simulink model "system_sim"  (R2015a)
settings: Solver=ode45  StartTime=0.0  StopTime=3600 *10  FixedStep=0.2  RelTol=0.001
values from neighbouring files (symbols this model uses):
  area = 1.2    [run_sim_auto.m]    (also in run_sim_test4.m = 2; sim_testing.m; wrkspc_no_1.mat; wrkspc_no_10.mat)
  Cd = 0.6    [run_sim_auto.m]    (also in run_sim_test4.m = 1; sim_testing.m; wrkspc_no_1.mat; wrkspc_no_10.mat)
  Crr = 0.005    [run_sim_test4.m]    (also in wrkspc_no_1.mat; wrkspc_no_10.mat; wrkspc_no_18.mat; wrkspc_no_22.mat)
  eff_vals = eff_data(:,2)    [run_sim_auto.m]    (also in wrkspc_no_1.mat = [5.2 10.3 15.5 20.6 25.8 31 36.1 41.3 46.4 51.6 56.8 61.9 ..; wrkspc_no_10.mat = [5.2 10.3 15.5 20.6 25.8 31 36.1 41.3 46.4 51.6 56.8 61.9 ..; wrkspc_no_18.mat = [5.2 10.3 15.5 20.6 25.8 31 36.1 41.3 46.4 51.6 56.8 61.9 ..; wrkspc_no_22.mat = [5.2 10.3 15.5 20.6 25.8 31 36.1 41.3 46.4 51.6 56.8 61.9 ..)
  end_x = x_in_m(length(x_in_m))    [run_sim_auto.m]    (also in run_sim_v2.m; wrkspc_no_1.mat = 44100; wrkspc_no_10.mat = 48084; wrkspc_no_18.mat = 8912)
  fmax = max_moving_force    [run_sim_auto.m]    (also in run_sim_v2.m; wrkspc_no_1.mat = 666.666666667; wrkspc_no_10.mat = 666.666666667; wrkspc_no_18.mat = 666.666666667)
  g = 9.81    [run_sim.m]    (also in run_sim_auto.m; run_sim_test.m; run_sim_test4.m; run_sim_v2.m)
  input_rpm_vals = eff_data(:,1)    [run_sim_auto.m]    (also in wrkspc_no_1.mat = [10 20 30 40 50 60 70 80 90 100 110 120 ... (35 elements, 35; wrkspc_no_10.mat = [10 20 30 40 50 60 70 80 90 100 110 120 ... (35 elements, 35; wrkspc_no_18.mat = [10 20 30 40 50 60 70 80 90 100 110 120 ... (35 elements, 35; wrkspc_no_22.mat = [10 20 30 40 50 60 70 80 90 100 110 120 ... (35 elements, 35)
  m = 210    [run_sim_auto.m]    (also in run_sim_test4.m = 150; sim_testing.m; wrkspc_no_1.mat; wrkspc_no_10.mat)
  rho_air = 1.225    [run_sim.m]    (also in run_sim_auto.m; run_sim_test.m; run_sim_test4.m; run_sim_v2.m)
  slope = target_speed_m_s/acc_time    [run_sim_auto.m]    (also in run_sim_v2.m; wrkspc_no_1.mat = 0.833333333333; wrkspc_no_10.mat = 0.833333333333; wrkspc_no_18.mat = 0.833333333333)
  target_speed_m_s = 4.16    [run_sim_test4.m]    (also in wrkspc_no_1.mat = 4.16666666667; wrkspc_no_10.mat = 4.16666666667; wrkspc_no_18.mat = 4.16666666667; wrkspc_no_22.mat = 4.16666666667)
  wheel_radius = 0.2538    [wrkspc_no_1.mat]    (also in wrkspc_no_10.mat; wrkspc_no_18.mat; wrkspc_no_22.mat)
libraries: simulink x1
settings Model: Creator=marco  LastModifiedBy=marco

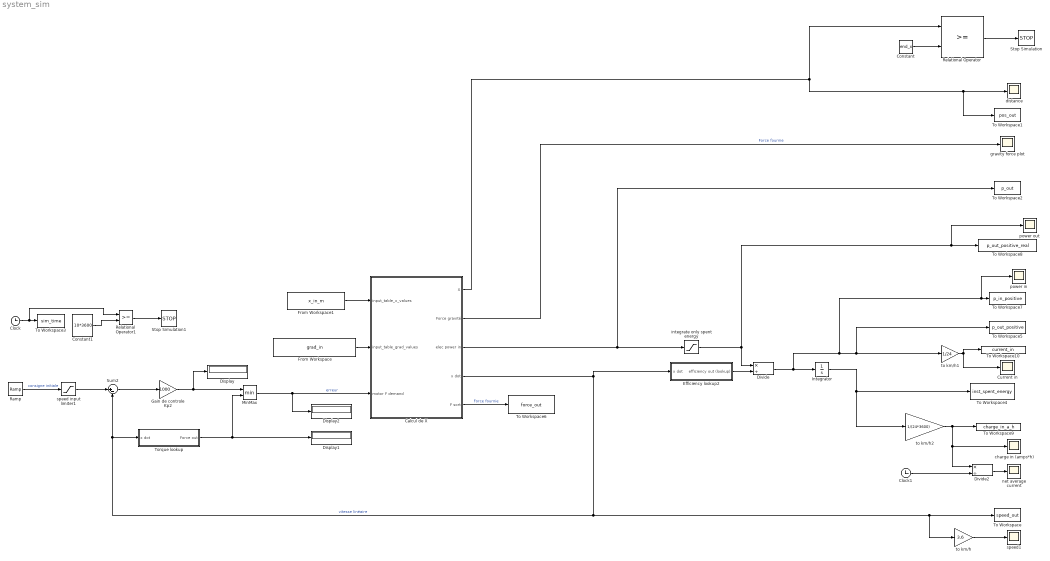
== system system_sim ==
  Calcul de X : Subsystem
  Clock : Clock
  Clock1 : Clock
  Constant : Constant  Value=end_x
  Constant1 : Constant  Value=10*3600
  Current in : Scope
      settings: TimeRange=10000  YMin=0  YMax=40  SaveName=ScopeData5  MaxDataPoints=scope_history*3
  Display : Display
  Display1 : Display
  Display2 : Display
  Divide : Product  Inputs=*/
  Divide2 : Product  Inputs=*/
  Efficiency lookup2 : Subsystem
  From Workspace : FromWorkspace  VariableName=grad_in  SampleTime=0
  From Workspace1 : FromWorkspace  VariableName=x_in_m  SampleTime=0
  Gain de controle Kp2 : Gain  Gain=1000
  Integrator : Integrator
  MinMax : MinMax  Inputs=2
  Ramp : simulink/Sources/Ramp  slope=slope  start=0  X0=0
  Relational Operator : RelationalOperator  OutDataTypeStr=boolean
  Relational Operator1 : RelationalOperator  OutDataTypeStr=boolean
  Stop Simulation : Stop
  Stop Simulation1 : Stop
  Sum2 : Sum  Inputs=|+-
  To Workspace : ToWorkspace  VariableName=speed_out  SampleTime=-1
      settings: Save2DSignal=2-D array (concatenate along first dimension)
  To Workspace1 : ToWorkspace  VariableName=pos_out  SampleTime=-1
      settings: Save2DSignal=2-D array (concatenate along first dimension)
  To Workspace10 : ToWorkspace  VariableName=current_in  SampleTime=-1
      settings: Save2DSignal=2-D array (concatenate along first dimension)
  To Workspace2 : ToWorkspace  VariableName=p_out  SampleTime=-1
      settings: Save2DSignal=2-D array (concatenate along first dimension)
  To Workspace3 : ToWorkspace  VariableName=sim_time  SampleTime=-1
      settings: Save2DSignal=2-D array (concatenate along first dimension)
  To Workspace4 : ToWorkspace  VariableName=inst_spent_energy  SampleTime=-1
      settings: Save2DSignal=2-D array (concatenate along first dimension)
  To Workspace5 : ToWorkspace  VariableName=p_out_positive  SampleTime=-1
      settings: Save2DSignal=2-D array (concatenate along first dimension)
  To Workspace6 : ToWorkspace  VariableName=force_out  SampleTime=-1
      settings: Save2DSignal=2-D array (concatenate along first dimension)
  To Workspace7 : ToWorkspace  VariableName=p_in_positive  SampleTime=-1
      settings: Save2DSignal=2-D array (concatenate along first dimension)
  To Workspace8 : ToWorkspace  VariableName=p_out_positive_real  SampleTime=-1
      settings: Save2DSignal=2-D array (concatenate along first dimension)
  To Workspace9 : ToWorkspace  VariableName=charge_in_a_h  SampleTime=-1
      settings: Save2DSignal=2-D array (concatenate along first dimension)
  Torque lookup : Subsystem
  charge in (amps*h) : Scope
      settings: TimeRange=30000  YMin=160000  YMax=300000  SaveName=ScopeData7  MaxDataPoints=scope_history *3
  distance : Scope
      settings: YMin=25000  YMax=52500  MaxDataPoints=scope_history
  gravity force plot : Scope
      settings: YMin=3.55  YMax=4.45  MaxDataPoints=scope_history
  integrate only spent energy : Saturate  UpperLimit=fmax*target_speed_m_s*8  LowerLimit=0
  net average current : Scope
      settings: TimeRange=10000  YMin=0  YMax=40  SaveName=ScopeData11  MaxDataPoints=scope_history*3
  power in : Scope
      settings: YMin=0  YMax=425  SaveName=powerin_scope  MaxDataPoints=scope_history*3
  power out : Scope
      settings: YMin=0  YMax=525  SaveName=powerin_scope1  MaxDataPoints=scope_history*3
  speed input limiter1 : Saturate  UpperLimit=target_speed_m_s  LowerLimit=0
  speed1 : Scope
      settings: YMin=7  YMax=15.5  SaveName=speed_kmh_scope  MaxDataPoints=scope_history*3
  to km/h : Gain  Gain=3.6
  to km/h1 : Gain  Gain=1/24
  to km/h2 : Gain  Gain=1/(24*3600)
  wires:
  From Workspace1/1 -> Calcul de X/1(input_table_x_values)
  From Workspace/1 -> Calcul de X/2(input_table_grad_values)
  MinMax/1 -> Calcul de X/3(motor F demand), Display2/1  "erreur"
  Calcul de X/1(X) -> To Workspace1/1, distance/1, Relational Operator/1
  Constant/1 -> Relational Operator/2
  Relational Operator/1 -> Stop Simulation/1
  Clock/1 -> Relational Operator1/1, To Workspace3/1
  Integrator/1 -> to km/h2/1, To Workspace4/1
  integrate only spent energy/1 -> Divide/1, power out/1, To Workspace8/1
  Calcul de X/3(elec power in) -> To Workspace2/1, integrate only spent energy/1
  Constant1/1 -> Relational Operator1/2
  Relational Operator1/1 -> Stop Simulation1/1
  to km/h/1 -> speed1/1
  Calcul de X/5(F sort) -> To Workspace6/1  "Force fournie"
  Ramp/1 -> speed input limiter1/1  "consigne initiale"
  Gain de controle Kp2/1 -> Display/1, MinMax/1
  Sum2/1 -> Gain de controle Kp2/1
  Efficiency lookup2/1(efficiency out (lookup)) -> Divide/2
  Divide/1 -> Integrator/1, power in/1, To Workspace7/1, to km/h1/1, To Workspace5/1
  Calcul de X/4(x dot) -> Sum2/2, Torque lookup/1(x dot), To Workspace/1, to km/h/1, Efficiency lookup2/1(x dot)  "vitesse linéaire"
  speed input limiter1/1 -> Sum2/1
  to km/h1/1 -> Current in/1, To Workspace10/1
  to km/h2/1 -> To Workspace9/1, Divide2/1, charge in (amps*h)/1
  Clock1/1 -> Divide2/2
  Divide2/1 -> net average current/1
  Calcul de X/2(Force gravité) -> gravity force plot/1  "Force fournie"
  Torque lookup/1(Force out) -> MinMax/2, Display1/1

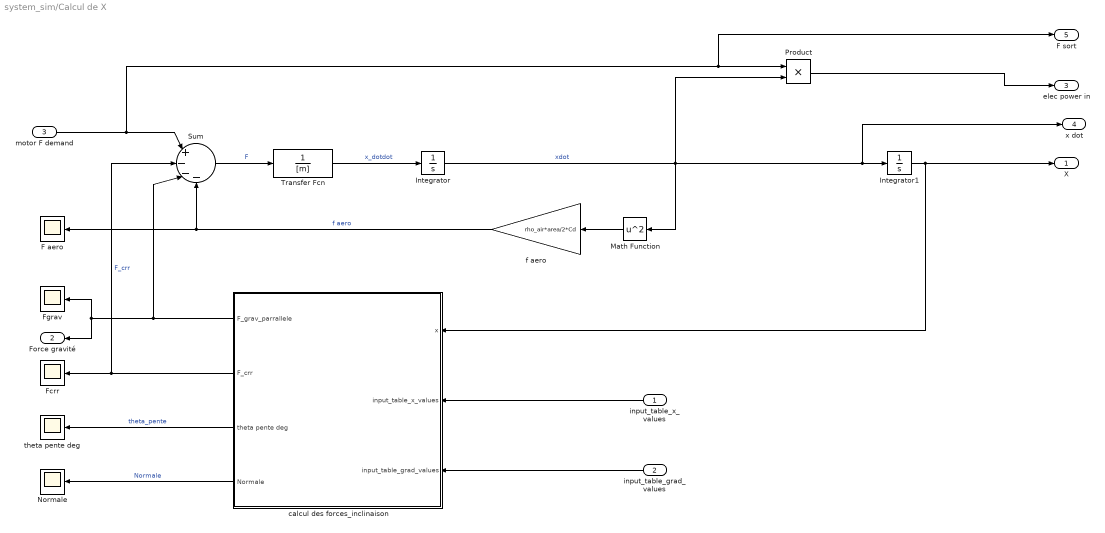
== system system_sim/Calcul de X ==
  input_table_x_values : Inport
  input_table_grad_values : Inport  Port=2
  motor F demand : Inport  Port=3
  F aero : Scope
      settings: SaveName=ScopeData14  MaxDataPoints=scope_history
  Fcrr : Scope
      settings: SaveName=ScopeData10  MaxDataPoints=scope_history
  Fgrav : Scope
      settings: YMin=-70  YMax=70  SaveName=ScopeData9  MaxDataPoints=scope_history*3
  Integrator : Integrator
  Integrator1 : Integrator
  Math Function : Math  Operator=square  SaturateOnIntegerOverflow=on
  Normale : Scope
      settings: SaveName=ScopeData2  MaxDataPoints=scope_history
  Product : Product
  Sum : Sum  Inputs=|+---
  Transfer Fcn : TransferFcn  Denominator=[m]
  calcul des forces_inclinaison : Subsystem
  f aero : Gain  Gain=rho_air*area/2*Cd
  "theta pente deg " : Scope
      settings: YMin=-15  YMax=17.5  SaveName=gradiant  MaxDataPoints=scope_history*3
  X : Outport
  Force gravité : Outport  Port=2
  elec power in : Outport  Port=3
  x dot : Outport  Port=4
  F sort : Outport  Port=5
  wires:
  Sum/1 -> Transfer Fcn/1  "F"
  Transfer Fcn/1 -> Integrator/1  "x_dotdot"
  Integrator/1 -> Math Function/1, Product/2, x dot/1, Integrator1/1  "xdot"
  f aero/1 -> F aero/1, Sum/4  "f aero"
  input_table_x_values/1 -> calcul des forces_inclinaison/2(input_table_x_values)
  input_table_grad_values/1 -> calcul des forces_inclinaison/3(input_table_grad_values)
  Math Function/1 -> f aero/1
  Integrator1/1 -> X/1, calcul des forces_inclinaison/1(x)
  calcul des forces_inclinaison/3(theta pente deg) -> "theta pente deg "/1  "theta_pente"
  calcul des forces_inclinaison/2(F_crr) -> Sum/2, Fcrr/1  "F_crr"
  calcul des forces_inclinaison/1(F_grav_parrallele) -> Sum/3, Force gravité/1, Fgrav/1
  calcul des forces_inclinaison/4(Normale) -> Normale/1  "Normale"
  Product/1 -> elec power in/1
  motor F demand/1 -> Sum/1, F sort/1, Product/1

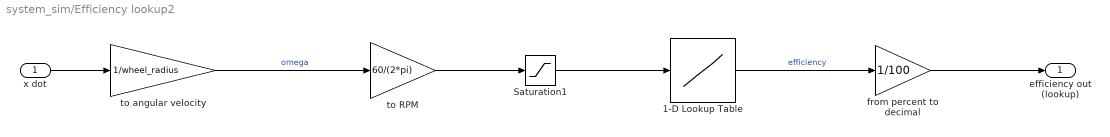
== system system_sim/Efficiency lookup2 ==
  x dot : Inport
  1-D Lookup Table : Lookup_n-D  NumberOfTableDimensions=1  BreakpointsForDimension1=input_rpm_vals  Table=eff_vals  InternalRulePriority=Speed  RndMeth=Simplest  InputSameDT=on
  Saturation1 : Saturate  UpperLimit=177  LowerLimit=10
  from percent to decimal : Gain  Gain=1/100
  to RPM : Gain  Gain=60/(2*pi)
  to angular velocity : Gain  Gain=1/wheel_radius
  efficiency out (lookup) : Outport
  wires:
  x dot/1 -> to angular velocity/1
  to angular velocity/1 -> to RPM/1  "omega"
  to RPM/1 -> Saturation1/1
  1-D Lookup Table/1 -> from percent to decimal/1  "efficiency"
  from percent to decimal/1 -> efficiency out (lookup)/1
  Saturation1/1 -> 1-D Lookup Table/1

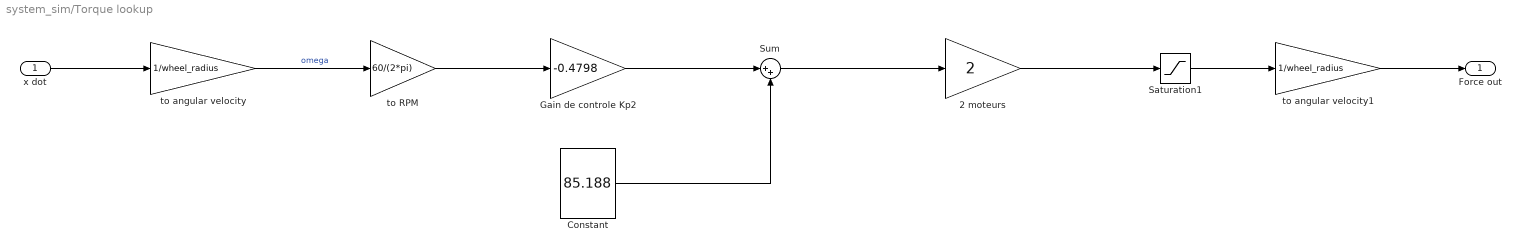
== system system_sim/Torque lookup ==
  x dot : Inport
  2 moteurs : Gain  Gain=2
  Constant : Constant  Value=85.188
  Gain de controle Kp2 : Gain  Gain=-0.4798
  Saturation1 : Saturate  UpperLimit=85.1*2  LowerLimit=-116*3
  Sum : Sum  Inputs=|++
  to RPM : Gain  Gain=60/(2*pi)
  to angular velocity : Gain  Gain=1/wheel_radius
  to angular velocity1 : Gain  Gain=1/wheel_radius
  Force out : Outport
  wires:
  x dot/1 -> to angular velocity/1
  to angular velocity/1 -> to RPM/1  "omega"
  Gain de controle Kp2/1 -> Sum/1
  to RPM/1 -> Gain de controle Kp2/1
  Sum/1 -> 2 moteurs/1
  Constant/1 -> Sum/2
  Saturation1/1 -> to angular velocity1/1
  to angular velocity1/1 -> Force out/1
  2 moteurs/1 -> Saturation1/1

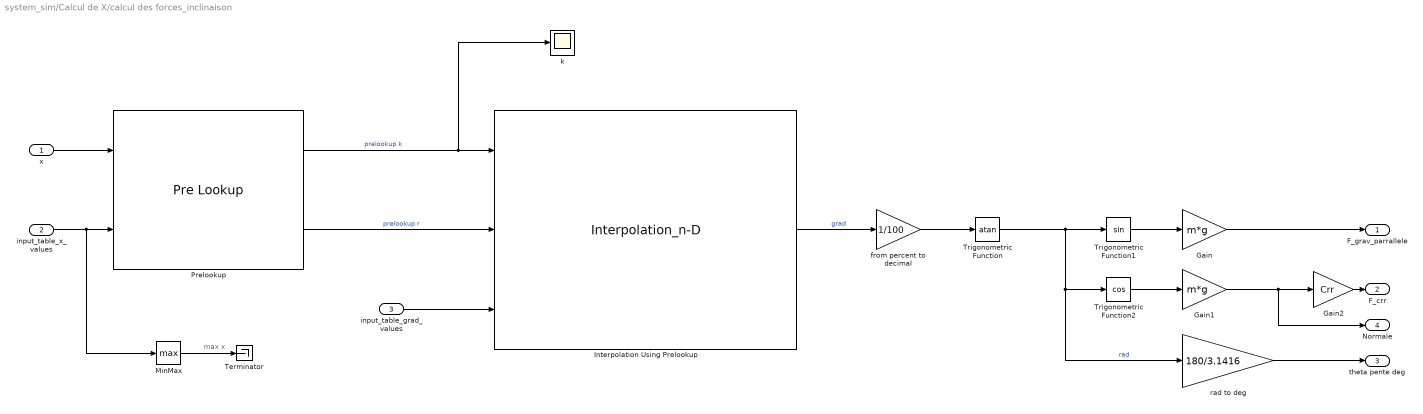
== system system_sim/Calcul de X/calcul des forces_inclinaison ==
  note: max x
  x : Inport
  input_table_x_values : Inport  Port=2
  input_table_grad_values : Inport  Port=3
  Gain : Gain  Gain=m*g
  Gain1 : Gain  Gain=m*g
  Gain2 : Gain  Gain=Crr
  Interpolation Using Prelookup : Interpolation_n-D  NumberOfTableDimensions=1  TableSource=Input port  InternalRulePriority=Speed
      settings: InputPortMap=u0,u1,p2
  MinMax : MinMax  Function=max
  Prelookup : PreLookup  BreakpointsDataSource=Input port  BreakpointsData=[10:10:110]  ExtrapMethod=Linear
      settings: InputPortMap=u0,p1
  Terminator : Terminator
  Trigonometric Function : Trigonometry  Operator=atan
  Trigonometric Function1 : Trigonometry
  Trigonometric Function2 : Trigonometry  Operator=cos
  from percent to decimal : Gain  Gain=1/100
  k : Scope
      settings: SaveName=ScopeData8  MaxDataPoints=scope_history
  rad to deg : Gain  Gain=180/3.1416
  F_grav_parrallele : Outport
  F_crr : Outport  Port=2
  theta pente deg : Outport  Port=3
  Normale : Outport  Port=4
  wires:
  x/1 -> Prelookup/1
  Interpolation Using Prelookup/1 -> from percent to decimal/1  "grad"
  Trigonometric Function1/1 -> Gain/1
  Trigonometric Function2/1 -> Gain1/1
  Gain1/1 -> Normale/1, Gain2/1
  Prelookup/1 -> k/1, Interpolation Using Prelookup/1  "prelookup k"
  Prelookup/2 -> Interpolation Using Prelookup/2  "prelookup r"
  input_table_grad_values/1 -> Interpolation Using Prelookup/3
  Trigonometric Function/1 -> rad to deg/1, Trigonometric Function2/1, Trigonometric Function1/1  "rad"
  from percent to decimal/1 -> Trigonometric Function/1
  input_table_x_values/1 -> MinMax/1, Prelookup/2
  Gain/1 -> F_grav_parrallele/1
  Gain2/1 -> F_crr/1
  rad to deg/1 -> theta pente deg/1
  MinMax/1 -> Terminator/1
